simulink model "M1_P2_B"  (R2023a)
settings: Solver=VariableStepAuto  StartTime=0.0  StopTime=2.5  RelTol=1e-3
undefined symbols (not defined in the file): f_eff, J_eff, Kb, Ktn, L, R
settings Model: Creator=azzam  LastModifiedBy=azzam

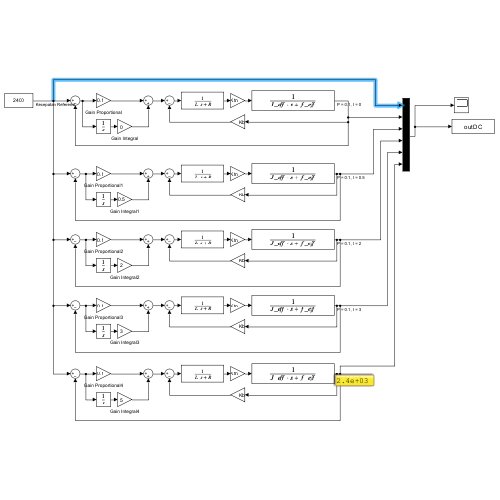
[thumbnail: Simulink's stored preview of the top-level diagram]
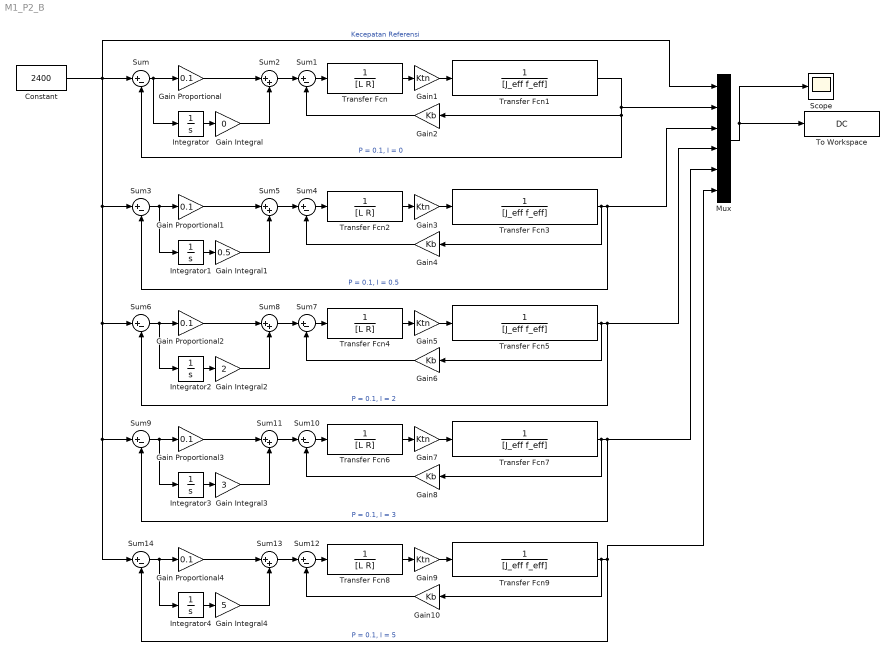
== system M1_P2_B ==
  Constant : Constant  Value=2400
  Gain Integral : Gain  Gain=0
  Gain Integral1 : Gain  Gain=0.5
  Gain Integral2 : Gain  Gain=2
  Gain Integral3 : Gain  Gain=3
  Gain Integral4 : Gain  Gain=5
  Gain Proportional{,1..4} (5 alike) : Gain  Gain=0.1
  Gain{1,3,5,7,9} (5 alike) : Gain  Gain=Ktn
  Gain{2,4,6,8,10} (5 alike) : Gain  Gain=Kb
  Integrator{,1..4} (5 alike) : Integrator
  Mux : Mux  Inputs=6
  Scope : Scope
  Sum{,1,3..4,6..7,9..10,12,14} (10 alike) : Sum  Inputs=|+-
  Sum{2,5,8,11,13} (5 alike) : Sum  Inputs=|++
  To Workspace : ToWorkspace  VariableName=DC  SaveFormat=Timeseries  SampleTime=-1
  Transfer Fcn{,2,4,6,8} (5 alike) : TransferFcn  Denominator=[L R]
  Transfer Fcn{1,3,5,7,9} (5 alike) : TransferFcn  Denominator=[J_eff f_eff]
  wires:
  Transfer Fcn/1 -> Gain1/1
  Sum/1 -> Integrator/1, Gain Proportional/1
  Gain2/1 -> Sum1/2
  Gain1/1 -> Transfer Fcn1/1
  Transfer Fcn1/1 -> Gain2/1, Sum/2, Mux/2  "P = 0.1, I = 0"
  Sum1/1 -> Transfer Fcn/1
  Mux/1 -> Scope/1, To Workspace/1
  Gain Proportional/1 -> Sum2/1
  Sum2/1 -> Sum1/1
  Integrator/1 -> Gain Integral/1
  Gain Integral/1 -> Sum2/2
  Sum5/1 -> Sum4/1
  Integrator1/1 -> Gain Integral1/1
  Gain Integral1/1 -> Sum5/2
  Sum3/1 -> Integrator1/1, Gain Proportional1/1
  Transfer Fcn2/1 -> Gain3/1
  Gain4/1 -> Sum4/2
  Transfer Fcn3/1 -> Sum3/2, Mux/3, Gain4/1  "P = 0.1, I = 0.5"
  Sum4/1 -> Transfer Fcn2/1
  Gain Proportional1/1 -> Sum5/1
  Gain3/1 -> Transfer Fcn3/1
  Gain6/1 -> Sum7/2
  Sum6/1 -> Integrator2/1, Gain Proportional2/1
  Sum7/1 -> Transfer Fcn4/1
  Gain5/1 -> Transfer Fcn5/1
  Gain Proportional2/1 -> Sum8/1
  Transfer Fcn4/1 -> Gain5/1
  Transfer Fcn5/1 -> Mux/4, Sum6/2, Gain6/1  "P = 0.1, I = 2"
  Sum8/1 -> Sum7/1
  Gain Integral2/1 -> Sum8/2
  Integrator2/1 -> Gain Integral2/1
  Transfer Fcn7/1 -> Mux/5, Sum9/2, Gain8/1  "P = 0.1, I = 3"
  Integrator3/1 -> Gain Integral3/1
  Sum11/1 -> Sum10/1
  Gain8/1 -> Sum10/2
  Gain7/1 -> Transfer Fcn7/1
  Gain Proportional3/1 -> Sum11/1
  Sum10/1 -> Transfer Fcn6/1
  Sum9/1 -> Integrator3/1, Gain Proportional3/1
  Gain Integral3/1 -> Sum11/2
  Transfer Fcn6/1 -> Gain7/1
  Constant/1 -> Sum14/1, Sum9/1, Sum6/1, Sum3/1, Mux/1, Sum/1  "Kecepatan Referensi"
  Transfer Fcn8/1 -> Gain9/1
  Sum12/1 -> Transfer Fcn8/1
  Sum13/1 -> Sum12/1
  Gain Integral4/1 -> Sum13/2
  Gain10/1 -> Sum12/2
  Transfer Fcn9/1 -> Mux/6, Sum14/2, Gain10/1  "P = 0.1, I = 5"
  Gain9/1 -> Transfer Fcn9/1
  Gain Proportional4/1 -> Sum13/1
  Sum14/1 -> Integrator4/1, Gain Proportional4/1
  Integrator4/1 -> Gain Integral4/1
